simulink model "single_dioderectifier"  (Simulink 7.5)
settings: Solver=ode23tb  StartTime=0.0  StopTime=0.1  MaxStep=1e-5  RelTol=1e-3
libraries: powerlib x29, powerlib_extras x7
settings Model: Creator=viswam  LastModifiedBy=placements
settings SolverCC: InitialStep=1e-6
settings OptimizationCC: InitFltsAndDblsToZero=on
settings DebuggingCC: SaveWithParameterizedLinksMsg=none  SignalResolutionControl=TryResolveAllWithWarning  MultiTaskDSMMsg=warning  MultiTaskCondExecSysMsg=none  StrictBusMsg=Warning
settings RTWCC: IncludeERTFirstTime=on
settings GRTTargetCC: TargetFcnLib=ansi_tfl_tmw.mat

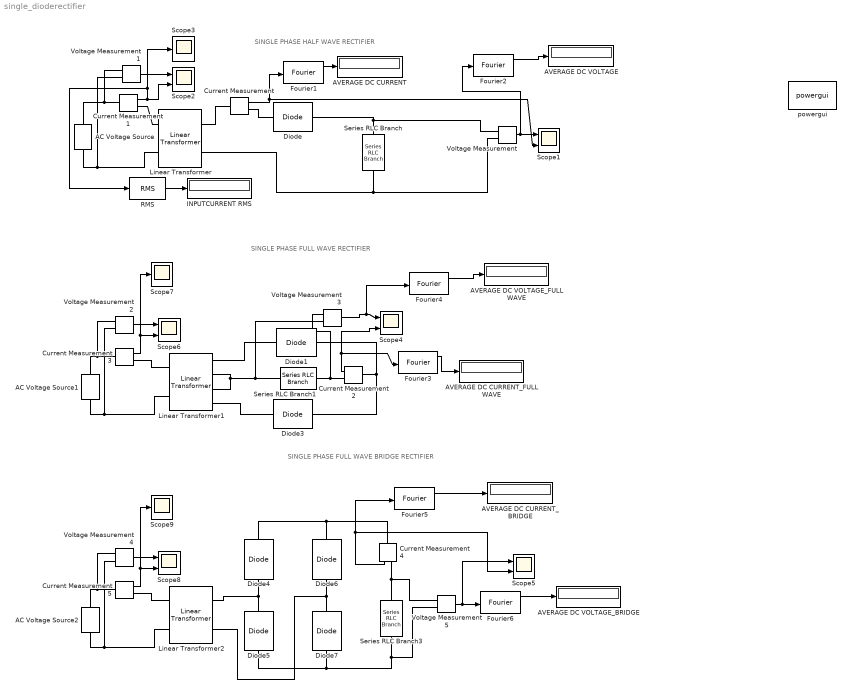
== system single_dioderectifier ==
  note: SINGLE PHASE HALF WAVE RECTIFIER
  note: SINGLE PHASE FULL WAVE RECTIFIER
  note: SINGLE PHASE FULL WAVE BRIDGE RECTIFIER
  AC Voltage Source : powerlib/Electrical Sources/AC Voltage Source  DialogController=POWERSYS.PowerSysDialog  SystemSampleTime=-1  Amplitude=230*sqrt(2)  Phase=0  Frequency=50  SampleTime=0  Measurements=None
  AC Voltage Source1 : powerlib/Electrical Sources/AC Voltage Source  DialogController=POWERSYS.PowerSysDialog  SystemSampleTime=-1  Amplitude=230*sqrt(2)  Phase=0  Frequency=50  SampleTime=0  Measurements=None
  AC Voltage Source2 : powerlib/Electrical Sources/AC Voltage Source  DialogController=POWERSYS.PowerSysDialog  SystemSampleTime=-1  Amplitude=230*sqrt(2)  Phase=0  Frequency=50  SampleTime=0  Measurements=None
  AVERAGE DC CURRENT : Display
  AVERAGE DC CURRENT_BRIDGE : Display
  AVERAGE DC CURRENT_FULL WAVE : Display
  AVERAGE DC VOLTAGE : Display
  AVERAGE DC VOLTAGE_BRIDGE : Display
  AVERAGE DC VOLTAGE_FULL WAVE : Display
  Current Measurement{,1..5} (6 alike) : powerlib/Measurements/Current Measurement  DialogController=POWERSYS.PowerSysDialog  SystemSampleTime=-1  PhasorSimulation=off  OutputType=Complex  PSBequivalent=0
  Diode{,1,3..7} (7 alike) : powerlib/Power Electronics/Diode  DialogController=POWERSYS.PowerSysDialog  SystemSampleTime=-1  Ron=0.001  Lon=0  Vf=0.8  IC=0  UseSnubber=off  Rs=500  Cs=250e-9  Measurements=off
  Fourier{1..6} (6 alike) : powerlib_extras/Measurements/Fourier  DialogController=POWERSYS.PowerSysDialog  SystemSampleTime=-1  f1=50  n=0
  INPUTCURRENT RMS : Display
  Linear Transformer : powerlib/Elements/Linear Transformer  DialogController=POWERSYS.PowerSysDialog  PhysicalDomain=powersysdomain  SubClassName=unknown  LeftPortType=p1  RightPortType=p1  LConnTagsString=a|b  RConnTagsString=A|B  UNITS=pu  NominalPower=[ 1000 50 ]  winding1=[ 230,0,0 ]  winding2=[ 230,0,0]  ThreeWindings=off  winding3=[ 60e3 0.005 0.02 ]  RmLm=[ inf,inf ]  Measurements=None  DataType=off
  Linear Transformer1 : powerlib/Elements/Linear Transformer  DialogController=POWERSYS.PowerSysDialog  PhysicalDomain=powersysdomain  SubClassName=unknown  LeftPortType=p1  RightPortType=p1  LConnTagsString=a|b  RConnTagsString=A|B|C|D  UNITS=pu  NominalPower=[ 1000 50 ]  winding1=[ 230,0,0 ]  winding2=[ 230,0,0]  ThreeWindings=on  winding3=[ 230,0,0]  RmLm=[ inf,inf ]  Measurements=None  DataType=off
  Linear Transformer2 : powerlib/Elements/Linear Transformer  DialogController=POWERSYS.PowerSysDialog  PhysicalDomain=powersysdomain  SubClassName=unknown  LeftPortType=p1  RightPortType=p1  LConnTagsString=a|b  RConnTagsString=A|B  UNITS=pu  NominalPower=[ 1000 50 ]  winding1=[ 230,0,0 ]  winding2=[ 230,0,0]  ThreeWindings=off  winding3=[ 230,0,0]  RmLm=[ inf,inf ]  Measurements=None  DataType=off
  RMS : powerlib_extras/Measurements/RMS  DialogController=POWERSYS.PowerSysDialog  SystemSampleTime=-1  f1=50
  Scope{1..2,4..6,8} (6 alike) : Scope  NumInputPorts=2
      Scope1 settings: TimeRange=240  YMin=-5~-5  YMax=5~5
      Scope2 settings: TimeRange=240  YMin=-5~-5  YMax=5~5  SaveName=ScopeData2
      Scope4 settings: TimeRange=0.1  YMin=-50~0  YMax=350~35
      Scope5 settings: TimeRange=0.1  YMin=0~19.5163  YMax=325~21.5707  SaveName=ScopeData4
      Scope6 settings: TimeRange=240  YMin=-5~-5  YMax=5~5  SaveName=ScopeData3
      Scope8 settings: TimeRange=240  YMin=-5~-5  YMax=5~5  SaveName=ScopeData5
  Scope3 : Scope
      settings: TimeRange=240  SaveName=INPUTCURRENTHALFWAVE
  Scope7 : Scope
      settings: TimeRange=240  SaveName=INPUTCURRENTFULLWAVE
  Scope9 : Scope
      settings: TimeRange=240  SaveName=INPUTCURRENTFULLWAVE1
  Series RLC Branch : powerlib/Elements/Series RLC Branch  DialogController=POWERSYS.PowerSysDialog  PhysicalDomain=powersysdomain  SubClassName=unknown  LeftPortType=p1  RightPortType=p1  LConnTagsString=__new0  RConnTagsString=__new0  BranchType=R  Resistance=10  Inductance=10e-3  SetiL0=off  InitialCurrent=0  Capacitance=1e-6  Setx0=off  InitialVoltage=0  Measurements=None
  Series RLC Branch1 : powerlib/Elements/Series RLC Branch  DialogController=POWERSYS.PowerSysDialog  PhysicalDomain=powersysdomain  SubClassName=unknown  LeftPortType=p1  RightPortType=p1  LConnTagsString=__new0  RConnTagsString=__new0  BranchType=R  Resistance=10  Inductance=1e-3  SetiL0=off  InitialCurrent=0  Capacitance=1e-6  Setx0=off  InitialVoltage=0  Measurements=None
  Series RLC Branch3 : powerlib/Elements/Series RLC Branch  DialogController=POWERSYS.PowerSysDialog  PhysicalDomain=powersysdomain  SubClassName=unknown  LeftPortType=p1  RightPortType=p1  LConnTagsString=__new0  RConnTagsString=__new0  BranchType=R  Resistance=10  Inductance=1e-3  SetiL0=off  InitialCurrent=0  Capacitance=1e-6  Setx0=off  InitialVoltage=0  Measurements=None
  Voltage Measurement{,1..5} (6 alike) : powerlib/Measurements/Voltage Measurement  DialogController=POWERSYS.PowerSysDialog  SystemSampleTime=-1  PhasorSimulation=off  OutputType=Complex  PSBequivalent=0
  powergui : powerlib/powergui  Priority=1  SystemSampleTime=-1  SimulationMode=Continuous  SampleTime=50e-6  frequency=60  SPID=off  DisableSnubberDevices=off  DisableRonSwitches=off  DisableVfSwitches=off  SwTol=0  Interpol=off  frequencyindice=50  echomessages=off  HookPort=off  DisplayEquations=off  FunctionMessages=off  EnableUseOfTLC=off  x0status=blocks  RestoreLinks=warning  ResistiveCurrentMeasurement=off  Frange=[0:2:500]  Ylog=off  Xlog=on  ShowGrid=off  save=off  variable=ZData  ZoomFFT=on  StartTime=0.0  cycles=1  DisplayStyle=1  fundamental=60  FreqAxis=off  MaxFrequency=1000  frequencyindicesteady=1  RmsSteady=1  display=off  Ts=0  methode=off
  wires:
  Current Measurement/1 -> Fourier1/1, Scope1/2
  Voltage Measurement1/1 -> Scope2/1
  Fourier2/1 -> AVERAGE DC VOLTAGE/1
  Fourier1/1 -> AVERAGE DC CURRENT/1
  Voltage Measurement/1 -> Scope1/1, Fourier2/1
  Current Measurement1/1 -> Scope2/2, Scope3/1, RMS/1
  RMS/1 -> INPUTCURRENT RMS/1
  Voltage Measurement3/1 -> Scope4/1, Fourier4/1
  Current Measurement2/1 -> Scope4/2, Fourier3/1
  Voltage Measurement2/1 -> Scope6/1
  Current Measurement3/1 -> Scope6/2, Scope7/1
  Fourier3/1 -> AVERAGE DC CURRENT_FULL WAVE/1
  Fourier4/1 -> AVERAGE DC VOLTAGE_FULL WAVE/1
  Voltage Measurement4/1 -> Scope8/1
  Current Measurement5/1 -> Scope9/1, Scope8/2
  Fourier5/1 -> AVERAGE DC CURRENT_BRIDGE/1
  Fourier6/1 -> AVERAGE DC VOLTAGE_BRIDGE/1
  Voltage Measurement5/1 -> Fourier6/1, Scope5/1
  Current Measurement4/1 -> Fourier5/1, Scope5/2
  connections:
  Voltage Measurement1/LConn1 -- AC Voltage Source/RConn1 -- Current Measurement1/LConn1
  AC Voltage Source/LConn1 -- Linear Transformer/LConn2 -- Voltage Measurement1/LConn2
  Current Measurement/LConn1 -- Linear Transformer/RConn1
  Linear Transformer/RConn2 -- Series RLC Branch/RConn1 -- Voltage Measurement/LConn2
  Diode/RConn1 -- Series RLC Branch/LConn1 -- Voltage Measurement/LConn1
  Current Measurement/RConn1 -- Diode/LConn1
  Current Measurement1/RConn1 -- Linear Transformer/LConn1
  Series RLC Branch1/RConn1 -- Linear Transformer1/RConn2 -- Linear Transformer1/RConn3 -- Voltage Measurement3/LConn2
  Linear Transformer1/RConn1 -- Diode1/LConn1
  Linear Transformer1/RConn4 -- Diode3/LConn1
  Current Measurement2/RConn1 -- Series RLC Branch1/LConn1 -- Voltage Measurement3/LConn1
  Diode1/RConn1 -- Current Measurement2/LConn1 -- Diode3/RConn1
  Current Measurement3/RConn1 -- Linear Transformer1/LConn1
  AC Voltage Source1/RConn1 -- Current Measurement3/LConn1 -- Voltage Measurement2/LConn1
  AC Voltage Source1/LConn1 -- Linear Transformer1/LConn2 -- Voltage Measurement2/LConn2
  AC Voltage Source2/RConn1 -- Voltage Measurement4/LConn1 -- Current Measurement5/LConn1
  AC Voltage Source2/LConn1 -- Voltage Measurement4/LConn2 -- Linear Transformer2/LConn2
  Current Measurement5/RConn1 -- Linear Transformer2/LConn1
  Diode5/RConn1 -- Diode4/LConn1 -- Linear Transformer2/RConn1
  Diode7/RConn1 -- Diode6/LConn1 -- Linear Transformer2/RConn2
  Diode4/RConn1 -- Diode6/RConn1 -- Current Measurement4/LConn1
  Diode5/LConn1 -- Diode7/LConn1 -- Series RLC Branch3/LConn1 -- Voltage Measurement5/LConn2
  Current Measurement4/RConn1 -- Series RLC Branch3/RConn1 -- Voltage Measurement5/LConn1
